simulink model "Simulink_ARMAX"  (R2020b)
settings: Solver=VariableStepAuto  StartTime=0.0  StopTime=3600  RelTol=1e-3
undefined symbols (not defined in the file): A, b, B, c, D, I, N, P, Ts
settings Model: Creator=jerem  LastModifiedBy=jerem
settings SolverCC: AlgebraicLoopSolver=LineSearch

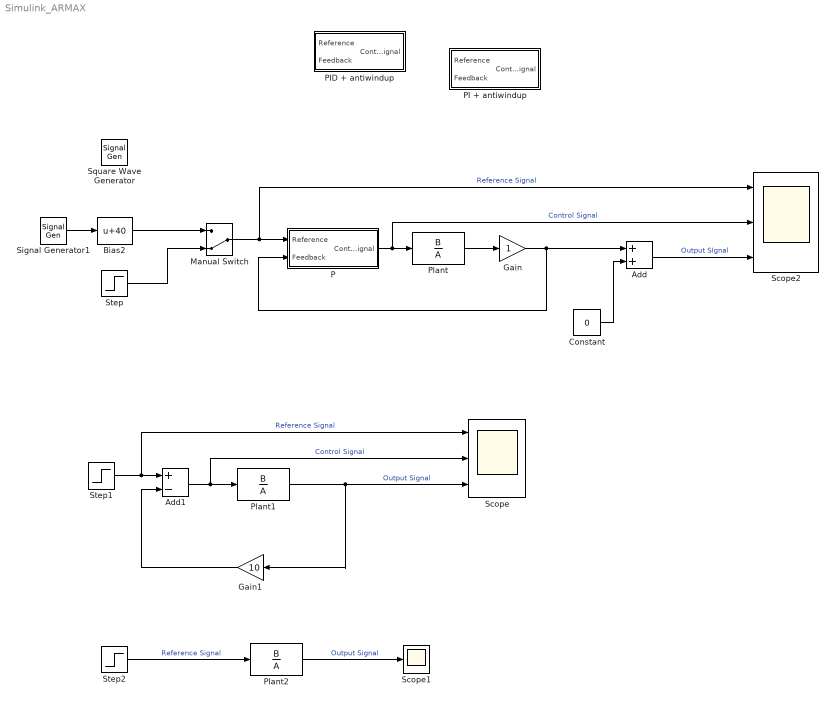
== system Simulink_ARMAX ==
  Add : Sum
  Add1 : Sum  Inputs=+-
  Bias2 : Bias  Bias=40
  Constant : Constant  Value=0
  Gain : Gain
  Gain1 : Gain  Gain=10
  Manual Switch : ManualSwitch  CurrentSetting=0
  P : Subsystem
  PI + antiwindup : Subsystem
  PID + antiwindup : Subsystem
  Plant : DiscreteTransferFcn  Numerator=B  Denominator=A  SampleTime=0.4
  Plant1 : DiscreteTransferFcn  Numerator=B  Denominator=A  SampleTime=0.4
  Plant2 : DiscreteTransferFcn  Numerator=B  Denominator=A  SampleTime=0.4
  Scope : Scope  NumInputPorts=3
  Scope1 : Scope
  Scope2 : Scope  NumInputPorts=3
  Signal Generator1 : SignalGenerator  WaveForm=square  Amplitude=40  Frequency=1/1800
  Square Wave Generator : SignalGenerator  WaveForm=square  Amplitude=40  Frequency=1/1800
  Step : Step  After=2  SampleTime=0.4
  Step1 : Step  After=0.1  SampleTime=0.4
  Step2 : Step  SampleTime=0.4
  wires:
  P/1(Control Signal) -> Scope2/2, Plant/1  "Control Signal"
  Signal Generator1/1 -> Bias2/1
  Plant/1 -> Gain/1
  Gain/1 -> P/2(Feedback), Add/1
  Manual Switch/1 -> P/1(Reference), Scope2/1  "Reference Signal"
  Bias2/1 -> Manual Switch/1
  Step/1 -> Manual Switch/2
  Add/1 -> Scope2/3  "Output SIgnal"
  Constant/1 -> Add/2
  Step1/1 -> Scope/1, Add1/1  "Reference Signal"
  Add1/1 -> Scope/2, Plant1/1  "Control Signal"
  Plant1/1 -> Gain1/1, Scope/3  "Output Signal"
  Step2/1 -> Plant2/1  "Reference Signal"
  Plant2/1 -> Scope1/1  "Output Signal"
  Gain1/1 -> Add1/2

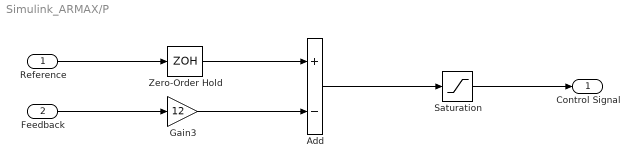
== system Simulink_ARMAX/P ==
  Reference : Inport
  Feedback : Inport  Port=2
  Add : Sum  Inputs=+-
  Gain3 : Gain  Gain=12
  Saturation : Saturate  UpperLimit=100  LowerLimit=0
  Zero-Order Hold : ZeroOrderHold  SampleTime=-1
  Control Signal : Outport
  wires:
  Reference/1 -> Zero-Order Hold/1
  Feedback/1 -> Gain3/1
  Gain3/1 -> Add/2
  Add/1 -> Saturation/1
  Saturation/1 -> Control Signal/1
  Zero-Order Hold/1 -> Add/1

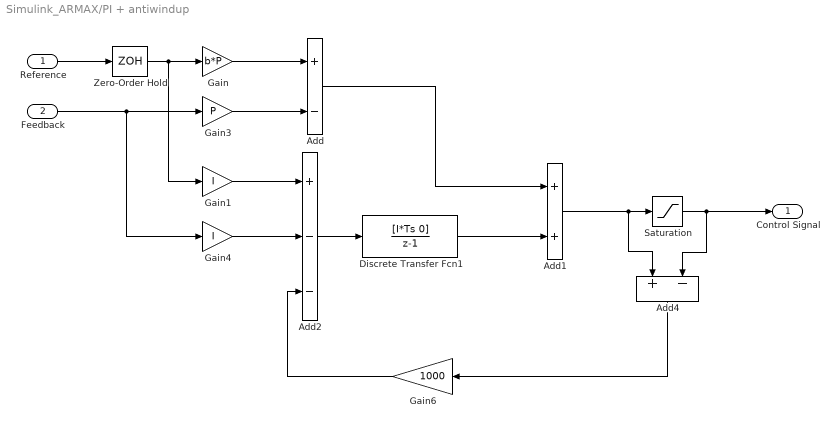
== system Simulink_ARMAX/PI + antiwindup ==
  Reference : Inport
  Feedback : Inport  Port=2
  Add : Sum  Inputs=+-
  Add1 : Sum
  Add2 : Sum  Inputs=+--
  Add4 : Sum  Inputs=+-
  Discrete Transfer Fcn1 : DiscreteTransferFcn  Numerator=[I*Ts 0]  Denominator=[1 -1]
  Gain : Gain  Gain=b*P
  Gain1 : Gain  Gain=I
  Gain3 : Gain  Gain=P
  Gain4 : Gain  Gain=I
  Gain6 : Gain  Gain=1000
  Saturation : Saturate  UpperLimit=100  LowerLimit=0
  Zero-Order Hold : ZeroOrderHold  SampleTime=-1
  Control Signal : Outport
  wires:
  Reference/1 -> Zero-Order Hold/1
  Zero-Order Hold/1 -> Gain1/1, Gain/1
  Gain/1 -> Add/1
  Feedback/1 -> Gain4/1, Gain3/1
  Gain3/1 -> Add/2
  Gain4/1 -> Add2/2
  Gain1/1 -> Add2/1
  Add2/1 -> Discrete Transfer Fcn1/1
  Add/1 -> Add1/1
  Discrete Transfer Fcn1/1 -> Add1/2
  Add1/1 -> Add4/1, Saturation/1
  Saturation/1 -> Control Signal/1, Add4/2
  Add4/1 -> Gain6/1
  Gain6/1 -> Add2/3

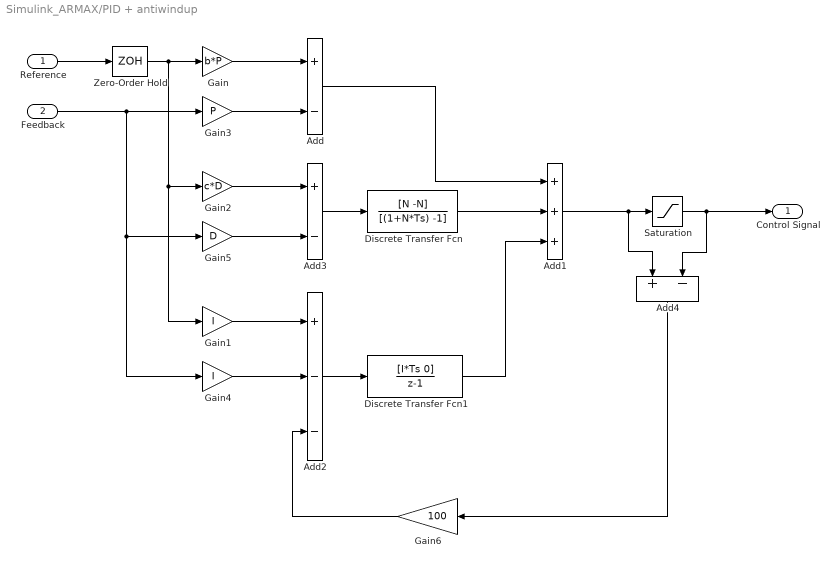
== system Simulink_ARMAX/PID + antiwindup ==
  Reference : Inport
  Feedback : Inport  Port=2
  Add : Sum  Inputs=+-
  Add1 : Sum  Inputs=+++
  Add2 : Sum  Inputs=+--
  Add3 : Sum  Inputs=+-
  Add4 : Sum  Inputs=+-
  Discrete Transfer Fcn : DiscreteTransferFcn  Numerator=[N -N]  Denominator=[(1+N*Ts) -1]
  Discrete Transfer Fcn1 : DiscreteTransferFcn  Numerator=[I*Ts 0]  Denominator=[1 -1]
  Gain : Gain  Gain=b*P
  Gain1 : Gain  Gain=I
  Gain2 : Gain  Gain=c*D
  Gain3 : Gain  Gain=P
  Gain4 : Gain  Gain=I
  Gain5 : Gain  Gain=D
  Gain6 : Gain  Gain=100
  Saturation : Saturate  UpperLimit=100  LowerLimit=0
  Zero-Order Hold : ZeroOrderHold  SampleTime=-1
  Control Signal : Outport
  wires:
  Reference/1 -> Zero-Order Hold/1
  Zero-Order Hold/1 -> Gain1/1, Gain2/1, Gain/1
  Gain/1 -> Add/1
  Feedback/1 -> Gain4/1, Gain5/1, Gain3/1
  Gain3/1 -> Add/2
  Gain4/1 -> Add2/2
  Gain2/1 -> Add3/1
  Gain5/1 -> Add3/2
  Gain1/1 -> Add2/1
  Add2/1 -> Discrete Transfer Fcn1/1
  Add3/1 -> Discrete Transfer Fcn/1
  Discrete Transfer Fcn/1 -> Add1/2
  Add/1 -> Add1/1
  Discrete Transfer Fcn1/1 -> Add1/3
  Add1/1 -> Add4/1, Saturation/1
  Saturation/1 -> Control Signal/1, Add4/2
  Add4/1 -> Gain6/1
  Gain6/1 -> Add2/3
